simulink model "siso_4_channel_teleop_discrete_tank_forcePos_noise"  (R2021a)
settings: Solver=FixedStepAuto  StartTime=0.0  StopTime=30  FixedStep=Ts  RelTol=1e-3
values from neighbouring files (symbols this model uses):
  A_kalman = [1 Ts ; 0 1 ]    [assignment7.m]
  alpha = 0.1    [assignment7.m]
  Amplitude = 1    [assignment7.m]
  Be = 10    [assignment7.m]
  beta = 0.01    [assignment7.m]
  Bh = 1.5    [assignment7.m]
  Bs = 20    [assignment7.m]
  C_kalman = [1 0]    [assignment7.m]
  delay = 20    [assignment7.m]
  Dh = 2    [assignment7.m]
  Dm = 0    [assignment7.m]
  Ds = 0    [assignment7.m]
  Fc = 0.1    [assignment7.m]
  Flp = 5    [assignment7.m]
  H0_master = 1    [assignment7.m]
  Hd = 1    [assignment7.m]
  Ih = 0    [assignment7.m]
  Jh = 0    [assignment7.m]
  k_h = 2    [assignment7.m]
  Ke = 200    [assignment7.m]
  Kh = 1    [assignment7.m]
  Ks = 25    [assignment7.m]
  Mm = 0.5    [assignment7.m]
  Ms = 2    [assignment7.m]
  noiseVariance = 0.00001    (= 1e-05)    [assignment7.m]
  R = 1    [assignment7.m]
  Ts = 0.001    [assignment7.m]
  xe = 0.65    [assignment7.m]
undefined symbols (not defined in the file or in its folder): B, D, Discrete, Time
libraries: simulink x2, ctrlSharedLib x2
settings Model: Creator=fabio  LastModifiedBy=fabio
settings DebuggingCC: UnderSpecifiedDimensionMsg=warning

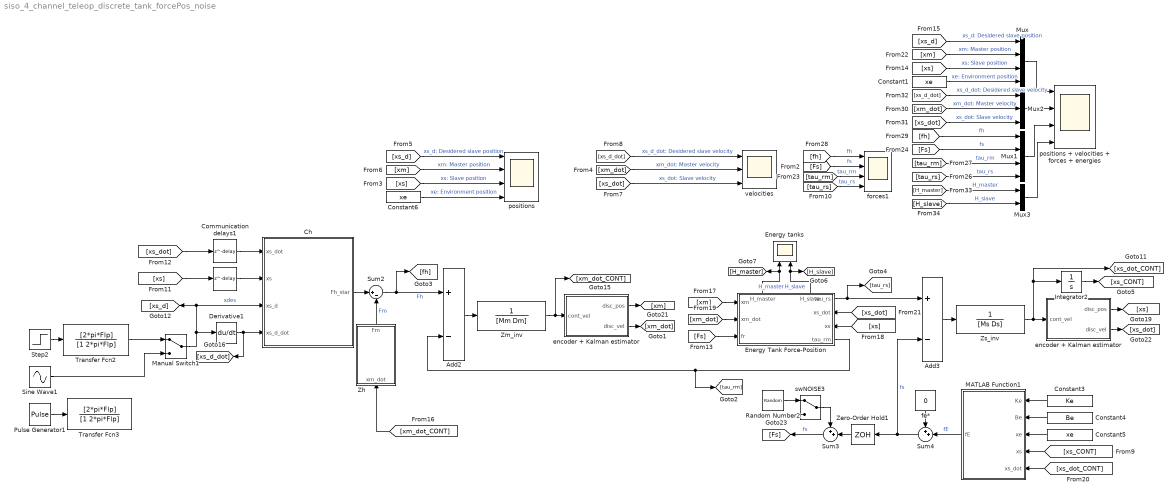
== system siso_4_channel_teleop_discrete_tank_forcePos_noise ==
  " " : Delay  DelayLength=delay  SampleTime=Ts
  Add2 : Sum  Inputs=+-
  Add3 : Sum  Inputs=+-
  Ch : Subsystem
  Communication delays1 : Delay  DelayLength=delay  SampleTime=Ts
  Constant1 : Constant  Value=xe
  Constant3 : Constant  Value=Ke
  Constant4 : Constant  Value=Be
  Constant5 : Constant  Value=xe
  Constant6 : Constant  Value=xe
  Derivative1 : Derivative
  Energy Tank Force-Position : Subsystem
      settings: PortSchema="{\"entries\":[{\"content\":{\"sides\":[{\"content\":{\"connectorIds\":[\"In1\",\"In2\",\"In3\"]},\"type\":\"ConnectorPlacement.EquallySpacedRectSide\",\"uuid\":\"f2b5b233-4bc9-48fa-8c02-3c8bfabc8edf\"},{\"content\":{\"connectorIds\":[\"Out1\",\"In4\",\"In5\",\"Out2\"],\"side\":\"RIGHT\"},\"type\":\"ConnectorPlacement.EquallySpacedRectSide\",\"uuid\":\"567bdcc6-c695-4210-9521-fb074471be82\"},{\"content\":{\"connectorIds\":[\"Out3\",\"Out4\"],\"side\":\"TOP\"},\"type\":\"ConnectorPlacement.EquallySpacedRectSide\",\"uuid\":\"1a36b9db-f8a2-44fb-9901-095b7ca2258a\"},{\"content\":{\"connectorIds\":[],\"side\":\"BOTTOM\"},\"type\":\"ConnectorPlacement.EquallySpacedRectSide\",\"uuid\":\"a909301a-5578-4141-9a94-8638dffcae66\"},{\"content\":{\"connectorIds\":[],\"side\":\"HIDDEN\"},\"type\":\"ConnectorPlacement.EquallySpacedRectSide\",\"uuid\":\"2e8b54c5-18c4-4c1b-a8a4-ee42e67d82c7\"}]},\"type\":\"ConnectorPlacement.EquallySpacedConnector\",\"uuid\":\"569d959e-ea5b-42c6-b188-2deb8683cad8\"}],\"packageUris\":[\"http://schema.mathworks.com/mf0/Connector/R2020b\"],\"version\":\"1.0\"}"
  Energy tanks : Scope  NumInputPorts=2
  Integrator2 : Integrator
  MATLAB Function1 : MATLAB Function  TreatAsAtomicUnit=on
  Manual Switch1 : ManualSwitch
  Mux : Mux
  Mux1 : Mux
  Mux2 : Mux  Inputs=3
  Mux3 : Mux  Inputs=2
  Pulse Generator1 : DiscretePulseGenerator  PulseType=Time based  Amplitude=Amplitude  PulseWidth=50  PhaseDelay=1
  Random Number2 : RandomNumber  Variance=noiseVariance  SampleTime=Ts
  Sine Wave1 : Sin  Amplitude=Amplitude  Frequency=Fc*2*pi  SampleTime=0
  Step2 : Step  After=Amplitude  SampleTime=0
  Sum2 : Sum  Inputs=|+-
  Sum3 : Sum  Inputs=++|
  Sum4 : Sum  Inputs=++|
  Transfer Fcn2 : TransferFcn  Numerator=[2*pi*Flp]  Denominator=[1 2*pi*Flp]
  Transfer Fcn3 : TransferFcn  Numerator=[2*pi*Flp]  Denominator=[1 2*pi*Flp]
  Zero-Order Hold1 : ZeroOrderHold  SampleTime=Ts
  Zh : Subsystem
  Zm_inv : TransferFcn  Numerator=[0 1]  Denominator=[Mm Dm]
  Zs_inv : TransferFcn  Numerator=[0 1]  Denominator=[Ms Ds]
  encoder + Kalman estimator : Subsystem
  "encoder + Kalman estimator " : Subsystem
  fe* : Constant  Value=0
  forces1 : Scope  NumInputPorts=4
  positions : Scope  NumInputPorts=4
  positions + velocities + forces + energies : Scope  NumInputPorts=4
  swNOISE3 : ManualSwitch
  velocities : Scope  NumInputPorts=3
  wires:
  [xs_d] -> positions/1  "xs_d: Desidered slave position"
  [xm] -> positions/2  "xm: Master position"
  [xs] -> positions/3  "xs: Slave position"
  [xm_dot] -> velocities/2  "xm_dot: Master velocity"
  [xs_dot] -> velocities/3  "xs_dot: Slave velocity"
  [xs_d_dot] -> velocities/1  "xs_d_dot: Desidered slave velocity"
  Constant6/1 -> positions/4  "xe: Environment position"
  [Fs] -> Energy Tank Force-Position/3(fr)
  Sum4/1 -> Zero-Order Hold1/1, Add3/2  "fs"
  [xs] -> " "/1
  [xs_dot_CONT] -> MATLAB Function1/5(xs_dot)
  [xm] -> Energy Tank Force-Position/1(xm)
  Integrator2/1 -> [xs_CONT]
  Add2/1 -> Zm_inv/1
  Zero-Order Hold1/1 -> Sum3/2
  [xm_dot_CONT] -> Zh/1(xm_dot)
  [xm_dot] -> Energy Tank Force-Position/2(xm_dot)
  Sum3/1 -> [Fs]  "fs"
  MATLAB Function1/1(fE) -> Sum4/2  "fE"
  Energy Tank Force-Position/2(tau_rm) -> [tau_rm], Add2/2
  " "/1 -> Ch/3(xs)
  Derivative1/1 -> Ch/1(xs_d_dot), [xs_d_dot]
  Zh/1(Fm) -> Sum2/2  "Fm"
  Add3/1 -> Zs_inv/1
  Constant3/1 -> MATLAB Function1/1(Ke)
  Constant4/1 -> MATLAB Function1/2(Be)
  [xs_dot] -> Communication delays1/1
  Communication delays1/1 -> Ch/4(xs_dot)
  Sum2/1 -> Add2/1, [fh]  "Fh"
  Zm_inv/1 -> encoder + Kalman estimator/1(cont_vel), [xm_dot_CONT]
  fe*/1 -> Sum4/1
  Ch/1(Fh_star) -> Sum2/1
  [xs_CONT] -> MATLAB Function1/4(xs)
  "encoder + Kalman estimator "/2(disc_vel) -> [xs_dot]
  Constant5/1 -> MATLAB Function1/3(xe)
  Zs_inv/1 -> "encoder + Kalman estimator "/1(cont_vel), [xs_dot_CONT], Integrator2/1
  "encoder + Kalman estimator "/1(disc_pos) -> [xs]
  encoder + Kalman estimator/2(disc_vel) -> [xm_dot]
  encoder + Kalman estimator/1(disc_pos) -> [xm]
  Manual Switch1/1 -> Ch/2(xs_d), [xs_d], Derivative1/1  "xdes"
  Step2/1 -> Transfer Fcn2/1
  Pulse Generator1/1 -> Transfer Fcn3/1
  Transfer Fcn2/1 -> Manual Switch1/1
  Sine Wave1/1 -> Manual Switch1/2
  [xs] -> Energy Tank Force-Position/5(xs)
  [xs_dot] -> Energy Tank Force-Position/4(xs_dot)
  Energy Tank Force-Position/1(tau_rs) -> [tau_rs], Add3/1
  Mux3/1 -> positions + velocities + forces + energies/4
  [xs_dot] -> Mux2/3  "xs_dot: Slave velocity"
  [xm_dot] -> Mux2/2  "xm_dot: Master velocity"
  Mux/1 -> positions + velocities + forces + energies/1
  [tau_rs] -> Mux1/4  "tau_rs"
  [xs_d_dot] -> Mux2/1  "xs_d_dot: Desidered slave velocity"
  [H_master] -> Mux3/1  "H_master"
  Constant1/1 -> Mux/4  "xe: Environment position"
  [xs] -> Mux/3  "xs: Slave position"
  [xm] -> Mux/2  "xm: Master position"
  [xs_d] -> Mux/1  "xs_d: Desidered slave position"
  Mux1/1 -> positions + velocities + forces + energies/3
  Mux2/1 -> positions + velocities + forces + energies/2
  [fh] -> Mux1/1  "fh"
  [tau_rm] -> Mux1/3  "tau_rm"
  [tau_rm] -> forces1/3  "tau_rm"
  [H_slave] -> Mux3/2  "H_slave"
  [tau_rs] -> forces1/4  "tau_rs"
  [Fs] -> forces1/2  "fs"
  [Fs] -> Mux1/2  "fs"
  [fh] -> forces1/1  "fh"
  Energy Tank Force-Position/4(H_slave) -> Energy tanks/2, [H_slave]  "H_slave"
  Energy Tank Force-Position/3(H_master) -> [H_master], Energy tanks/1  "H_master"
  swNOISE3/1 -> Sum3/1
  Random Number2/1 -> swNOISE3/1

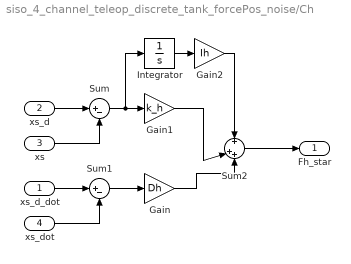
== system siso_4_channel_teleop_discrete_tank_forcePos_noise/Ch ==
  xs_d_dot : Inport
  xs_d : Inport  Port=2
  xs : Inport  Port=3
  xs_dot : Inport  Port=4
  Gain : Gain  Gain=Dh
  Gain1 : Gain  Gain=k_h
  Gain2 : Gain  Gain=Ih
  Integrator : Integrator
  Sum : Sum  Inputs=|+-
  Sum1 : Sum  Inputs=|+-
  Sum2 : Sum  Inputs=+|++
  Fh_star : Outport
  wires:
  Gain1/1 -> Sum2/2
  Sum2/1 -> Fh_star/1
  xs_d/1 -> Sum/1
  xs/1 -> Sum/2
  Sum/1 -> Integrator/1, Gain1/1
  xs_dot/1 -> Sum1/2
  Sum1/1 -> Gain/1
  Gain/1 -> Sum2/3
  xs_d_dot/1 -> Sum1/1
  Integrator/1 -> Gain2/1
  Gain2/1 -> Sum2/1

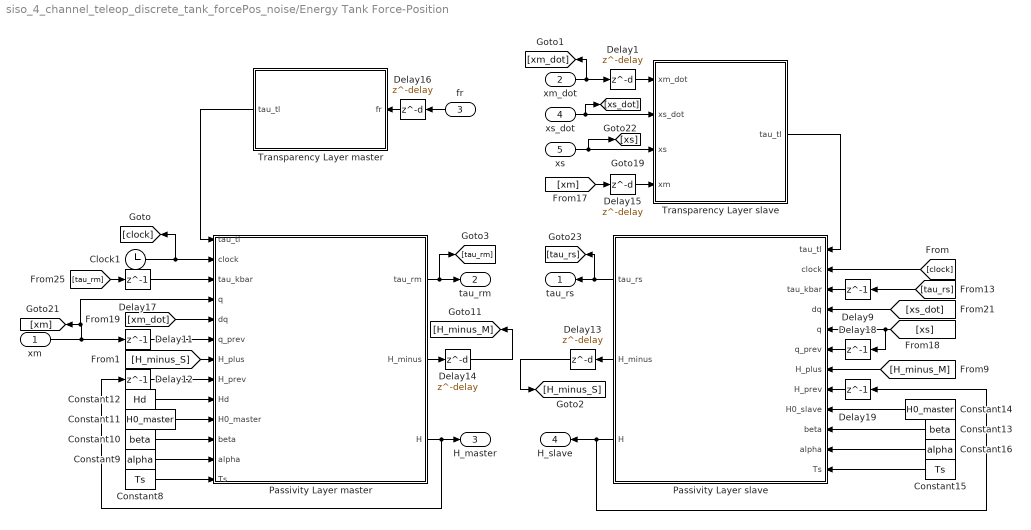
== system siso_4_channel_teleop_discrete_tank_forcePos_noise/Energy Tank Force-Position ==
  xm : Inport
  xm_dot : Inport  Port=2
  fr : Inport  Port=3
  xs_dot : Inport  Port=4
  xs : Inport  Port=5
  Clock1 : Clock
  Constant10 : Constant  Value=beta
  Constant11 : Constant  Value=H0_master
  Constant12 : Constant  Value=Hd
  Constant13 : Constant  Value=beta
  Constant14 : Constant  Value=H0_master
  Constant15 : Constant  Value=Ts
  Constant16 : Constant  Value=alpha
  Constant8 : Constant  Value=Ts
  Constant9 : Constant  Value=alpha
  Delay{1,13..16} (5 alike) : Delay  DelayLength=delay  SampleTime=Ts
  Delay{9,11..12,17..19} (6 alike) : Delay  DelayLength=1  SampleTime=Ts
  Passivity Layer master : MATLAB Function  TreatAsAtomicUnit=on
  Passivity Layer slave : MATLAB Function  TreatAsAtomicUnit=on
  Transparency Layer master : Subsystem
  Transparency Layer slave : Subsystem
  tau_rs : Outport
  tau_rm : Outport  Port=2
  H_master : Outport  Port=3
  H_slave : Outport  Port=4
  wires:
  xm_dot/1 -> [xm_dot], Delay1/1
  Delay1/1 -> Transparency Layer slave/1(xm_dot)
  Constant8/1 -> Passivity Layer master/13(Ts)
  Constant9/1 -> Passivity Layer master/12(alpha)
  Constant10/1 -> Passivity Layer master/11(beta)
  Constant12/1 -> Passivity Layer master/9(Hd)
  Constant11/1 -> Passivity Layer master/10(H0_master)
  Passivity Layer master/3(H) -> Delay12/1, H_master/1
  Delay12/1 -> Passivity Layer master/8(H_prev)
  Clock1/1 -> [clock], Passivity Layer master/2(clock)
  Delay11/1 -> Passivity Layer master/6(q_prev)
  Passivity Layer master/2(H_minus) -> Delay14/1
  Passivity Layer slave/2(H_minus) -> Delay13/1
  fr/1 -> Delay16/1
  Delay16/1 -> Transparency Layer master/1(fr)
  Transparency Layer master/1(tau_tl) -> Passivity Layer master/1(tau_tl)
  Passivity Layer master/1(tau_rm) -> [tau_rm], tau_rm/1
  Passivity Layer slave/1(tau_rs) -> [tau_rs], tau_rs/1
  Passivity Layer slave/3(H) -> Delay19/1, H_slave/1
  Transparency Layer slave/1(tau_tl) -> Passivity Layer slave/1(tau_tl)
  xs_dot/1 -> [xs_dot], Transparency Layer slave/2(xs_dot)
  Delay9/1 -> Passivity Layer slave/3(tau_kbar)
  [clock] -> Passivity Layer slave/2(clock)
  Delay15/1 -> Transparency Layer slave/4(xm)
  [xm] -> Delay15/1
  [xm_dot] -> Passivity Layer master/5(dq)
  Delay17/1 -> Passivity Layer master/3(tau_kbar)
  xm/1 -> Passivity Layer master/4(q), [xm], Delay11/1
  [tau_rm] -> Delay17/1
  xs/1 -> [xs], Transparency Layer slave/3(xs)
  [xs_dot] -> Passivity Layer slave/4(dq)
  [xs] -> Delay18/1, Passivity Layer slave/5(q)
  [tau_rs] -> Delay9/1
  Delay18/1 -> Passivity Layer slave/6(q_prev)
  Delay19/1 -> Passivity Layer slave/8(H_prev)
  Constant14/1 -> Passivity Layer slave/9(H0_slave)
  Constant15/1 -> Passivity Layer slave/12(Ts)
  Constant16/1 -> Passivity Layer slave/11(alpha)
  Constant13/1 -> Passivity Layer slave/10(beta)
  Delay14/1 -> [H_minus_M]
  Delay13/1 -> [H_minus_S]
  [H_minus_M] -> Passivity Layer slave/7(H_plus)
  [H_minus_S] -> Passivity Layer master/7(H_plus)

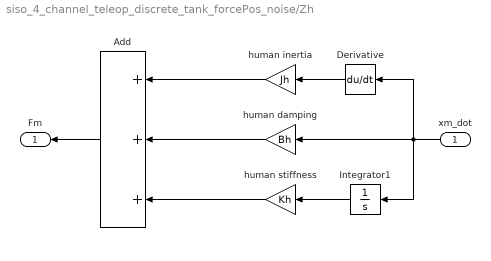
== system siso_4_channel_teleop_discrete_tank_forcePos_noise/Zh ==
  xm_dot : Inport
  Add : Sum  Inputs=+++
  Derivative : Derivative
  Integrator1 : Integrator
  human damping : Gain  Gain=Bh
  human inertia : Gain  Gain=Jh
  human stiffness : Gain  Gain=Kh
  Fm : Outport
  wires:
  Add/1 -> Fm/1
  human stiffness/1 -> Add/3
  human damping/1 -> Add/2
  Integrator1/1 -> human stiffness/1
  xm_dot/1 -> Derivative/1, Integrator1/1, human damping/1
  human inertia/1 -> Add/1
  Derivative/1 -> human inertia/1

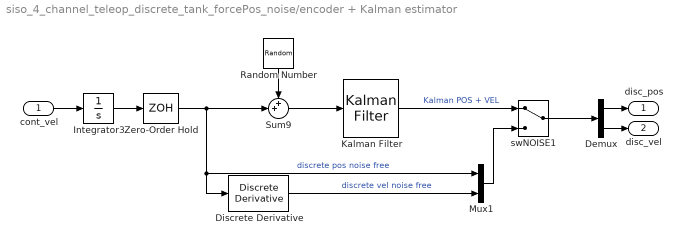
== system siso_4_channel_teleop_discrete_tank_forcePos_noise/encoder + Kalman estimator ==
  cont_vel : Inport
  Demux : Demux  Outputs=2
  Discrete Derivative : simulink/Discrete/Discrete Derivative  gainval=1.0  ICPrevScaledInput=0.0  OutMin=[]  OutMax=[]  OutDataType=fixdt(1, 16)  OutScaling=2^-10  DoSatur=off
  Integrator3 : Integrator
  Kalman Filter : ctrlSharedLib/Kalman Filter  TimeDomain=Discrete-Time  UseCurrentEstimator=on  ModelSource=Individual A, B, C, D matrices  ModelSourceVariable=sys  A=A_kalman  B=B  C=C_kalman  D=D  NumberOfStates=2  NumberOfInputs=2  NumberOfOutputs=2  InitialEstimateSource=Dialog  X0=0  P0=10  UseK=off  UseGH=off  NumberOfProcessNoiseInputs=2  G=1  TimeInvariantG=on  H=0  TimeInvariantH=on  Q=Q_master  TimeInvariantQ=on  R=R  TimeInvariantR=on  N=0  TimeInvariantN=on  AddInputPort=off  AddEnablePort=off  OutputEstimatedY=off  OutputP=off  Ts=Ts
  Mux1 : Mux  Inputs=2
  Random Number : RandomNumber  Variance=noiseVariance  SampleTime=Ts
  Sum9 : Sum  Inputs=++|
  Zero-Order Hold : ZeroOrderHold  SampleTime=Ts
  swNOISE1 : ManualSwitch
  disc_pos : Outport
  disc_vel : Outport  Port=2
  wires:
  Integrator3/1 -> Zero-Order Hold/1
  cont_vel/1 -> Integrator3/1
  Random Number/1 -> Sum9/1
  Zero-Order Hold/1 -> Discrete Derivative/1, Mux1/1, Sum9/2  "discrete pos noise free"
  Sum9/1 -> Kalman Filter/1
  Kalman Filter/1 -> swNOISE1/1  "Kalman POS + VEL"
  swNOISE1/1 -> Demux/1
  Demux/1 -> disc_pos/1
  Demux/2 -> disc_vel/1
  Discrete Derivative/1 -> Mux1/2  "discrete vel noise free"
  Mux1/1 -> swNOISE1/2

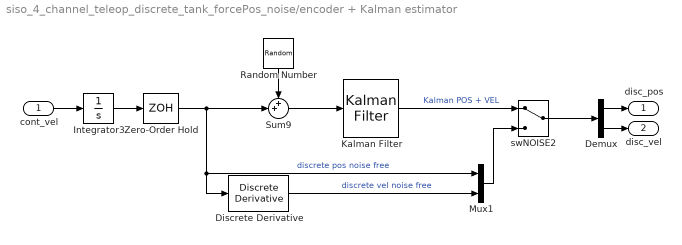
== system siso_4_channel_teleop_discrete_tank_forcePos_noise/encoder + Kalman estimator  ==
  cont_vel : Inport
  Demux : Demux  Outputs=2
  Discrete Derivative : simulink/Discrete/Discrete Derivative  gainval=1.0  ICPrevScaledInput=0.0  OutMin=[]  OutMax=[]  OutDataType=fixdt(1, 16)  OutScaling=2^-10  DoSatur=off
  Integrator3 : Integrator
  Kalman Filter : ctrlSharedLib/Kalman Filter  TimeDomain=Discrete-Time  UseCurrentEstimator=on  ModelSource=Individual A, B, C, D matrices  ModelSourceVariable=sys  A=A_kalman  B=B  C=C_kalman  D=D  NumberOfStates=2  NumberOfInputs=2  NumberOfOutputs=2  InitialEstimateSource=Dialog  X0=0  P0=10  UseK=off  UseGH=off  NumberOfProcessNoiseInputs=2  G=1  TimeInvariantG=on  H=0  TimeInvariantH=on  Q=Q_master  TimeInvariantQ=on  R=R  TimeInvariantR=on  N=0  TimeInvariantN=on  AddInputPort=off  AddEnablePort=off  OutputEstimatedY=off  OutputP=off  Ts=Ts
  Mux1 : Mux  Inputs=2
  Random Number : RandomNumber  Variance=noiseVariance  SampleTime=Ts
  Sum9 : Sum  Inputs=++|
  Zero-Order Hold : ZeroOrderHold  SampleTime=Ts
  swNOISE2 : ManualSwitch
  disc_pos : Outport
  disc_vel : Outport  Port=2
  wires:
  Integrator3/1 -> Zero-Order Hold/1
  cont_vel/1 -> Integrator3/1
  Random Number/1 -> Sum9/1
  Zero-Order Hold/1 -> Discrete Derivative/1, Mux1/1, Sum9/2  "discrete pos noise free"
  Sum9/1 -> Kalman Filter/1
  Kalman Filter/1 -> swNOISE2/1  "Kalman POS + VEL"
  swNOISE2/1 -> Demux/1
  Demux/1 -> disc_pos/1
  Demux/2 -> disc_vel/1
  Discrete Derivative/1 -> Mux1/2  "discrete vel noise free"
  Mux1/1 -> swNOISE2/2

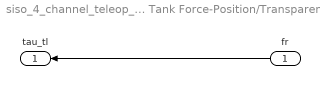
== system siso_4_channel_teleop_discrete_tank_forcePos_noise/Energy Tank Force-Position/Transparency Layer master ==
  fr : Inport
  tau_tl : Outport
  wires:
  fr/1 -> tau_tl/1

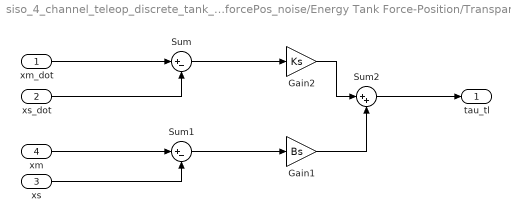
== system siso_4_channel_teleop_discrete_tank_forcePos_noise/Energy Tank Force-Position/Transparency Layer slave ==
  xm_dot : Inport
  xs_dot : Inport  Port=2
  xs : Inport  Port=3
  xm : Inport  Port=4
  Gain1 : Gain  Gain=Bs
  Gain2 : Gain  Gain=Ks
  Sum : Sum  Inputs=|+-
  Sum1 : Sum  Inputs=|+-
  Sum2 : Sum  Inputs=|++
  tau_tl : Outport
  wires:
  Sum/1 -> Gain2/1
  Sum2/1 -> tau_tl/1
  xs_dot/1 -> Sum/2
  Sum1/1 -> Gain1/1
  xm_dot/1 -> Sum/1
  Gain2/1 -> Sum2/1
  Gain1/1 -> Sum2/2
  xm/1 -> Sum1/1
  xs/1 -> Sum1/2

== matlab function siso_4_channel_teleop_discrete_tank_forcePos_noise/Energy Tank Force-Position/Passivity Layer slave ==
  data: tau_tl input; clock input; tau_rs output; H_minus output; H output; tau_kbar input; dq input; q input; q_prev input; H_plus input; H_prev input; H0_slave input; beta input; alpha input; Ts input
function [tau_rs,H_minus, H] = passivity_layer_slave(tau_tl, clock, tau_kbar, dq, q, q_prev, H_plus, H_prev, H0_slave, beta, alpha, Ts)
    %Initialization
    if clock == 0 %initialization
        H_prev = H0_slave;
        tau_kbar = 0; 
    end
    
    %Compute energy exchange
    deltaQ = q - q_prev;
    deltaH = tau_kbar * deltaQ;
    H = H_prev + H_plus - deltaH;

    %Comput maximum allowable torque
    if H <= 0 
        tau_max1 = 0;
    else
        tau_max1 = tau_tl;
    end

    if abs(dq) < 0.0001
        dq_temp = sign(dq)*0.0001; %impose dq this small to avoid infinity torque
        tau_max2 =  H/(dq_temp*Ts);
    else
        tau_max2 =  H/(dq*Ts);
    end 
    
    
    %Compute tau_rs
    tau_max = abs (min( tau_max1, tau_max2 ));
    tau_rs = sign(tau_tl)*min( abs(tau_tl), tau_max);

    %System sends an energy packet if possible
    if (H > 0)
        H_minus = beta*H;
        H = H - H_minus; 
    else
        H_minus = 0;
    end
end

== matlab function siso_4_channel_teleop_discrete_tank_forcePos_noise/Energy Tank Force-Position/Passivity Layer master ==
  data: tau_tl input; clock input; tau_rm output; H_minus output; tau_kbar input; q input; dq input; q_prev input; H_plus input; H_prev input; Hd input; H0_master input; beta input; alpha input; Ts input; H output
function [tau_rm, H_minus, H] = passivity_layer_master(tau_tl, clock, tau_kbar, q, dq, q_prev, H_plus, H_prev, Hd, H0_master, beta, alpha, Ts)
    %Initialization
    if clock == 0 %initialization
        H_prev = H0_master;
        tau_kbar = 0; 
    end
    
    %Compute energy exchange
    deltaQ = q - q_prev;
    deltaH = tau_kbar * deltaQ;
    H = H_prev + H_plus - deltaH;

    %Comput maximum allowable torque
    if H <= 0 
        tau_max1 = 0;
    else
        tau_max1 = tau_tl;
    end

    if abs(dq) < 0.0001
        dq_temp = sign(dq)*0.0001; %impose dq this small to avoid infinity torque
        tau_max2 =  H/(dq_temp*Ts);
    else
        tau_max2 =  H/(dq*Ts);
    end
   
    
    %Compute tau_rm
    tau_max = abs(min( tau_max1, tau_max2 ));
    tau_rm = sign(tau_tl)*min( abs(tau_tl), tau_max);

    %Tank level controller (only master)
    if(H < Hd)
       d = alpha*(Hd - H);
       tau_TLC = -d*dq;
       tau_rm = tau_rm + tau_TLC;
    end
    
    %System sends an energy packet if possible
    if (H > 0)
        H_minus = beta*H;
        H = H - H_minus; 
    else
        H_minus = 0;
    end
end

== matlab function siso_4_channel_teleop_discrete_tank_forcePos_noise/MATLAB Function1 ==
  data: Ke input; fE output; Be input; xe input; xs input; xs_dot input
function fE = environment(Ke, Be, xe, xs, xs_dot)
    if xs > xe
        fE = Ke*(xs - xe) + Be*xs_dot;
    else
        fE = 0;
    end
end
